simulink model "missle"  (R2021b)
settings: Solver=VariableStepAuto  StartTime=0.0  StopTime=1  MaxStep=1e-3  RelTol=1e-5
libraries: slpidlib x1
settings Model: Creator=Administrator  LastModifiedBy=Administrator

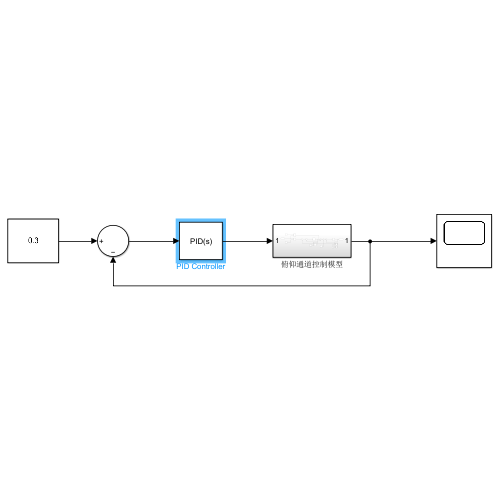
[thumbnail: Simulink's stored preview of the top-level diagram]
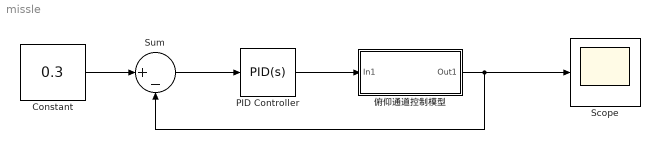
== system missle ==
  Constant : Constant  Value=0.3
  PID Controller : slpidlib/PID Controller  Controller=PID  Form=Parallel  TimeDomain=Continuous-time  UseExternalTs=off  SampleTime=-1  IntegratorMethod=Forward Euler  FilterMethod=Forward Euler  ControllerParametersSource=internal  P=-0.3  I=-30  D=-0.3  UseFilter=on  N=100  TunerSelectOption=Transfer Function Based (PID Tuner App)  InitialConditionSource=internal  InitialConditionForIntegrator=0  InitialConditionForFilter=0  DifferentiatorICPrevScaledInput=0  ExternalReset=none  TrackingMode=off  Kt=1  LimitOutput=off  SatLimitsSource=internal  UpperSaturationLimit=inf  LowerSaturationLimit=-inf  LinearizeAsGain=on  AntiWindupMode=none  Kb=1  POutMin=[]  POutMax=[]  IOutMin=[]  IOutMax=[]  DOutMin=[]  DOutMax=[]  NOutMin=[]  NOutMax=[]  SumOutMin=[]  SumOutMax=[]  SaturationOutMin=[]  SaturationOutMax=[]  PParamMin=[]  PParamMax=[]  IParamMin=[]  IParamMax=[]  DParamMin=[]  DParamMax=[]  NParamMin=[]  NParamMax=[]  KbParamMin=[]  KbParamMax=[]  KtParamMin=[]  KtParamMax=[]  KbOutMin=[]  KbOutMax=[]  KtOutMin=[]  KtOutMax=[]  IntegratorOutMin=[]  IntegratorOutMax=[]  FilterOutMin=[]  FilterOutMax=[]  SumI1OutMin=[]  SumI1OutMax=[]  SumI2OutMin=[]  SumI2OutMax=[]  SumI3OutMin=[]  SumI3OutMax=[]  SumI4OutMin=[]  SumI4OutMax=[]  SumDOutMin=[]  SumDOutMax=[]  DifferentiatorOutMin=[]  DifferentiatorOutMax=[]  FilterDiffOutCoefMin=[]  FilterDiffOutCoefMax=[]  ReciprocalOutMin=[]  ReciprocalOutMax=[]  SumDenOutMin=[]  SumDenOutMax=[]  SumNumOutMin=[]  SumNumOutMax=[]  DivideOutMin=[]  DivideOutMax=[]  UdiffTsProdOutMin=[]  UdiffTsProdOutMax=[]  NTsProdOutMin=[]  NTsProdOutMax=[]  UintegralTsProdOutMin=[]  UintegralTsProdOutMax=[]  UngainTsProdOutMin=[]  UngainTsProdOutMax=[]  IntegratorContinuousStateAttributes=''  IntegratorStateMustResolveToSignalObject=off  IntegratorRTWStateStorageClass=Auto  FilterContinuousStateAttributes=''  FilterStateMustResolveToSignalObject=off  FilterRTWStateStorageClass=Auto  ParallelPVariant=InternalParameters  IdealPVariant=Disabled  IVariant=InternalParameters  DVariant=InternalParameters  IntegratorVariant=Continuous  SatVariant=Disabled  AWVariant=Passthrough  PCopyVariant=Disabled  TRVariant=Disabled  FdbkBlocksVariant=Forward  IdealPFdbkVariant=Disabled  SatFdbkVariant=Disabled  DerivativeFilterVariant=ContFilter  NVariant=InternalParameters  NCopyVariant=Disabled  FilterICVariant=InternalICsFilter  IntegratorICVariant=InternalICs  ExternalResetVariant=Disabled  TRSumVariant=Passthrough  SumFdbkVariant=Disabled  SumVariant=Sum_PID  TsampFilterVariant=InternalTs  TsampNgainVariant=Passthrough  TsampIntegralVariant=Passthrough  ExternalSaturationOutDataTypeStr=Inherit: Same as second input
  Scope : Scope
  Sum : Sum  Inputs=|+-
  俯仰通道控制模型 : Subsystem
  wires:
  Sum/1 -> PID Controller/1
  Constant/1 -> Sum/1
  俯仰通道控制模型/1(Out1) -> Sum/2, Scope/1
  PID Controller/1 -> 俯仰通道控制模型/1(In1)

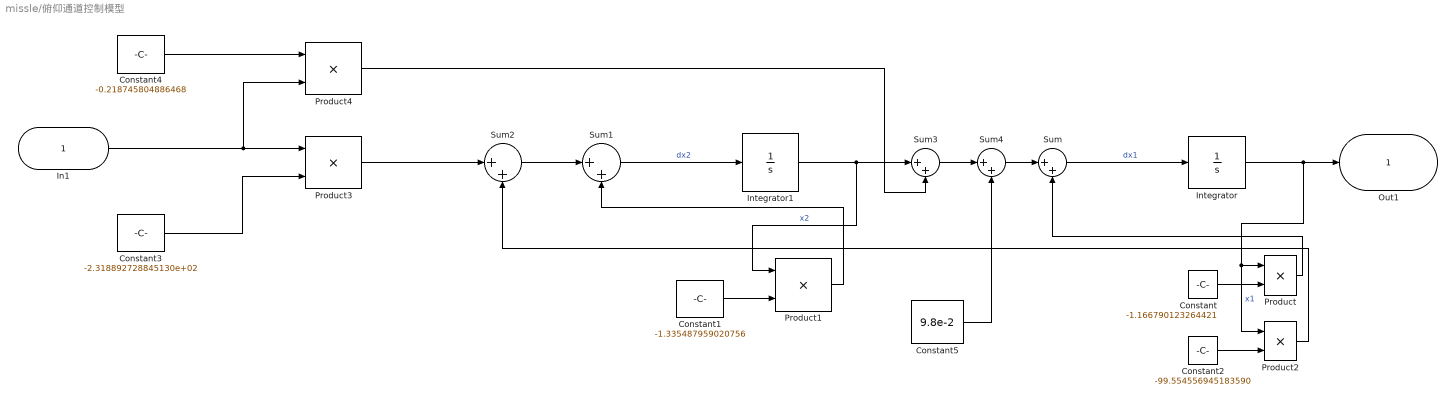
== system missle/俯仰通道控制模型 ==
  In1 : Inport
  Constant : Constant  Value=-1.166790123264421
  Constant1 : Constant  Value=-1.335487959020756
  Constant2 : Constant  Value=-99.554556945183590
  Constant3 : Constant  Value=-2.318892728845130e+02
  Constant4 : Constant  Value=-0.218745804886468
  Constant5 : Constant  Value=9.8e-2
  Integrator : Integrator
  Integrator1 : Integrator
  Product{,1..4} (5 alike) : Product
  Sum{,1..4} (5 alike) : Sum  Inputs=|++
  Out1 : Outport
  wires:
  In1/1 -> Product4/2, Product3/1
  Constant5/1 -> Sum4/2
  Constant2/1 -> Product2/2
  Sum4/1 -> Sum/1
  Constant4/1 -> Product4/1
  Integrator1/1 -> Sum3/1, Product1/1  "x2"
  Product2/1 -> Sum2/2
  Product4/1 -> Sum3/2
  Constant/1 -> Product/2
  Product1/1 -> Sum1/2
  Integrator/1 -> Out1/1, Product2/1, Product/1  "x1"
  Product3/1 -> Sum2/1
  Sum3/1 -> Sum4/1
  Constant1/1 -> Product1/2
  Sum2/1 -> Sum1/1
  Constant3/1 -> Product3/2
  Sum1/1 -> Integrator1/1  "dx2"
  Sum/1 -> Integrator/1  "dx1"
  Product/1 -> Sum/2
